simulink model "Closed_loop_Response"  (R2020a)
settings: Solver=VariableStepAuto  StartTime=0.0  StopTime=10  RelTol=1e-3
model workspace (MAT data in the model file):
  L = 1
  d = 0.3
settings Model: Creator=jgrou  LastModifiedBy=jgrou

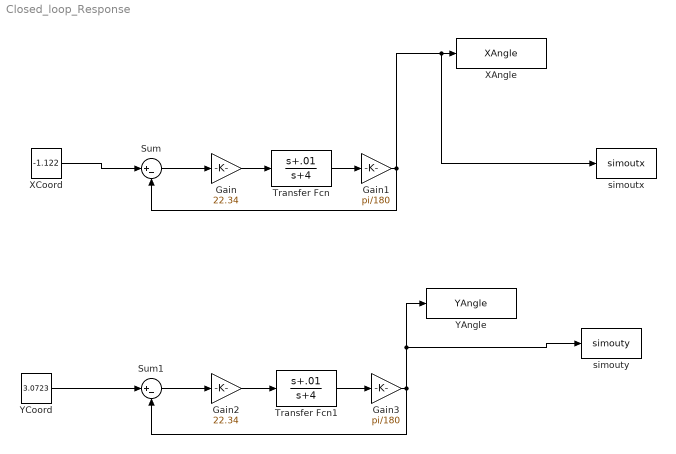
== system Closed_loop_Response ==
  Gain : Gain  Gain=22.34
  Gain1 : Gain  Gain=pi/180
  Gain2 : Gain  Gain=22.34
  Gain3 : Gain  Gain=pi/180
  Sum : Sum  Inputs=|+-
  Sum1 : Sum  Inputs=|+-
  Transfer Fcn : TransferFcn  Numerator=[1 .01]  Denominator=[1 4]
  Transfer Fcn1 : TransferFcn  Numerator=[1 .01]  Denominator=[1 4]
  XAngle : ToWorkspace  VariableName=XAngle  SaveFormat=Timeseries  SampleTime=-1
  XCoord : Constant  Value=-1.122
  YAngle : ToWorkspace  VariableName=YAngle  SaveFormat=Timeseries  SampleTime=-1
  YCoord : Constant  Value=3.0723
  simoutx : ToWorkspace  VariableName=simoutx  SaveFormat=Timeseries  SampleTime=-1
  simouty : ToWorkspace  VariableName=simouty  SaveFormat=Timeseries  SampleTime=-1
  wires:
  Sum/1 -> Gain/1
  Gain/1 -> Transfer Fcn/1
  Gain1/1 -> Sum/2, simoutx/1, XAngle/1
  Transfer Fcn/1 -> Gain1/1
  Gain3/1 -> Sum1/2, simouty/1, YAngle/1
  Transfer Fcn1/1 -> Gain3/1
  Sum1/1 -> Gain2/1
  Gain2/1 -> Transfer Fcn1/1
  XCoord/1 -> Sum/1
  YCoord/1 -> Sum1/1
